simulink model "project_simu"  (R2019a)
settings: Solver=VariableStepAuto  StartTime=0.0  StopTime=1  RelTol=1e-3
values from neighbouring files (symbols this model uses):
  banks = 1e6*banks_data    [project.m]
  f = Filters/mean(Filters)    [project.m]
  lines = lines_data    [project.m]
  loads = zeros(10,2)    [project.m]
  m = 2    [project.m]
libraries: powerlib x87, powerlib_meascontrol x1, sps_avr x1
(part 1 of 2)
settings Model: OrderedModelArguments=off  Creator=jedevisscher  LastModifiedBy=dimit
settings SolverCC: ZeroCrossAlgorithm=Adaptive
settings DataIOCC: ExternalInput=out.S5  ReturnWorkspaceOutputs=off
settings DebuggingCC: IgnoredZcDiagnostic=none  UnconnectedInputMsg=none  UnconnectedOutputMsg=none  UnconnectedLineMsg=none
settings SimscapeCC: SimscapeLogType=all  SimscapeLogSimulationStatistics=on  SimscapeLogToSDI=on  SimscapeLogOpenViewer=on

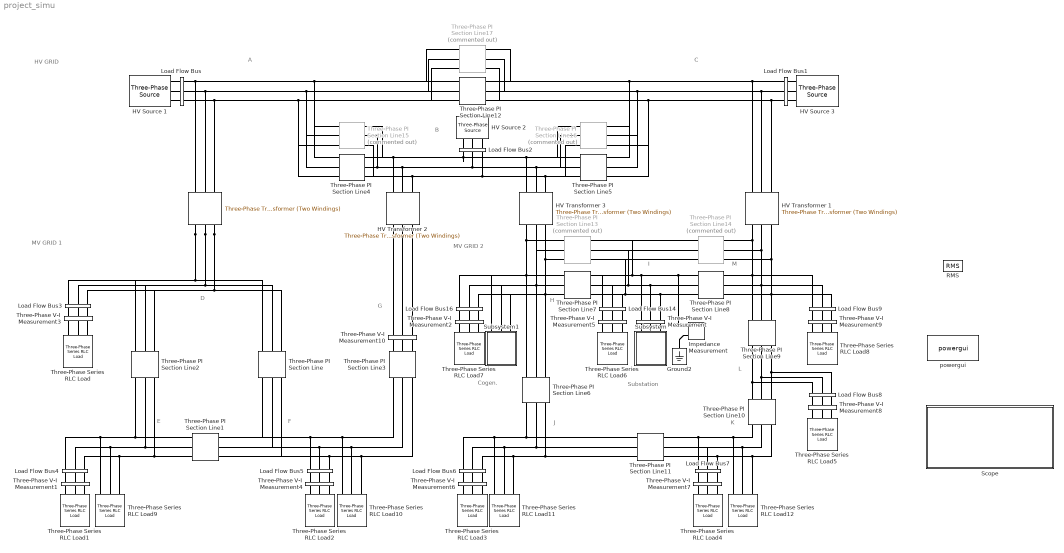
== system project_simu ==
  note: A
  note: B
  note: C
  note: D
  note: E
  note: F
  note: G
  note: H
  note: I
  note: J
  note: K
  note: L
  note: M
  note: HV GRID
  note: MV GRID 1
  note: MV GRID 2
  note: Substation
  note: Cogen.
  " " : powerlib/Elements/Three-Phase Transformer (Two Windings)  Winding1Connection=Yg  Winding2Connection=Yg  CoreType=Three single-phase transformers  SetSaturation=off  Hysteresis=off  DataFile='hysteresis'  SetInitialFlux=off  Measurements=None  UNITS=pu  NominalPower=[ 100e6 , 50 ]  Winding1=[220e3 0.002 0.08]  Winding2=[70e3 0.002 0.08]  Rm=500  Lm=500  L0=0.5  Saturation=[0 0;0.0024 1.2;0.99998 1.52]  InitialFluxes=[ 0.8 , -0.8 , 0.7 ]  BreakLoop=off  DiscreteSolver=Trapezoidal iterative  DataType=off  TransfoNumber=1
      settings: SourceProductName=Simscape Electrical
  Ground2 : powerlib/Elements/Ground  LConnTagsString=a
      settings: SourceProductName=Simscape Electrical
  HV Source 1 : powerlib/Electrical Sources/Three-Phase Source  InternalConnection=Yg  VoltagePhases=off  Voltage=220e3  PhaseAngle=0  Voltage_phases=[ 1.00409 1.00409 1.00409]*127017  PhaseAngles_phases=[ 1.18424 -118.816 121.184]  Frequency=50  NonIdealSource=on  SpecifyImpedance=on  Resistance=0  Inductance=0  ShortCircuitLevel=10e9  BaseVoltage=220e3  XRratio=7  BusType=swing  Pref=10e3  Qref=0  Prefabc=[3333.33 3333.33 3333.33]  Qrefabc=[0 0 0]  Qmin=-inf  Qmax=inf
      settings: SourceProductName=Simscape Electrical
  HV Source 2 : powerlib/Electrical Sources/Three-Phase Source  InternalConnection=Yg  VoltagePhases=off  Voltage=220e3  PhaseAngle=0  Voltage_phases=[ 1.01 1.01 1.01]*127017  PhaseAngles_phases=[ -2.01012 -122.01 117.99]  Frequency=50  NonIdealSource=on  SpecifyImpedance=on  Resistance=0  Inductance=0  ShortCircuitLevel=5e9  BaseVoltage=220e3  XRratio=6  BusType=PV  Pref=10e3  Qref=0  Prefabc=[3333.33 3333.33 3333.33]  Qrefabc=[0 0 0]  Qmin=-inf  Qmax=inf
      settings: SourceProductName=Simscape Electrical
  HV Source 3 : powerlib/Electrical Sources/Three-Phase Source  InternalConnection=Yg  VoltagePhases=off  Voltage=220e3  PhaseAngle=0  Voltage_phases=[ 1.01287 1.01287 1.01287]*127017  PhaseAngles_phases=[ -2.11617 -122.116 117.884]  Frequency=50  NonIdealSource=on  SpecifyImpedance=on  Resistance=0  Inductance=0  ShortCircuitLevel=3.5e9  BaseVoltage=220e3  XRratio=6  BusType=PV  Pref=10e3  Qref=0  Prefabc=[3333.33 3333.33 3333.33]  Qrefabc=[0 0 0]  Qmin=-inf  Qmax=inf
      settings: SourceProductName=Simscape Electrical
  HV Transformer 1 : powerlib/Elements/Three-Phase Transformer (Two Windings)  Winding1Connection=Yg  Winding2Connection=Yg  CoreType=Three single-phase transformers  SetSaturation=off  Hysteresis=off  DataFile='hysteresis'  SetInitialFlux=off  Measurements=None  UNITS=pu  NominalPower=[ 220e6 , 50 ]  Winding1=[220e3 0.001 0.1]  Winding2=[70e3 0.001 0.1]  Rm=500  Lm=500  L0=0.5  Saturation=[0 0;0.0024 1.2;0.99998 1.52]  InitialFluxes=[ 0.8 , -0.8 , 0.7 ]  BreakLoop=off  DiscreteSolver=Trapezoidal iterative  DataType=off  TransfoNumber=1
      settings: SourceProductName=Simscape Electrical
  HV Transformer 2 : powerlib/Elements/Three-Phase Transformer (Two Windings)  Winding1Connection=Yg  Winding2Connection=Yg  CoreType=Three single-phase transformers  SetSaturation=off  Hysteresis=off  DataFile='hysteresis'  SetInitialFlux=off  Measurements=None  UNITS=pu  NominalPower=[ 100e6 , 50 ]  Winding1=[220e3 0.002 0.075]  Winding2=[70e3 0.002 0.075]  Rm=500  Lm=500  L0=0.5  Saturation=[0 0;0.0024 1.2;0.99998 1.52]  InitialFluxes=[ 0.8 , -0.8 , 0.7 ]  BreakLoop=off  DiscreteSolver=Trapezoidal iterative  DataType=off  TransfoNumber=1
      settings: SourceProductName=Simscape Electrical
  HV Transformer 3 : powerlib/Elements/Three-Phase Transformer (Two Windings)  Winding1Connection=Yg  Winding2Connection=Yg  CoreType=Three single-phase transformers  SetSaturation=off  Hysteresis=off  DataFile='hysteresis'  SetInitialFlux=off  Measurements=None  UNITS=pu  NominalPower=[ 220e6 , 50 ]  Winding1=[220e3 0.001 0.1]  Winding2=[70e3 0.001 0.1]  Rm=500  Lm=500  L0=0.5  Saturation=[0 0;0.0024 1.2;0.99998 1.52]  InitialFluxes=[ 0.8 , -0.8 , 0.7 ]  BreakLoop=off  DiscreteSolver=Trapezoidal iterative  DataType=off  TransfoNumber=1
      settings: SourceProductName=Simscape Electrical
  Impedance Measurement : powerlib/Measurements/Impedance Measurement  LConnTagsString=+|-  Factor=1
      settings: SourceProductName=Simscape Electrical  SourceProductBaseCode=PS
  Load Flow Bus : powerlib/Measurements/Load Flow Bus  LConnTagsString=a|b|c  RConnTagsString=a|b|c  Phases=ABC  Connectors=on both sides  ID=BUS_A  Vbase=220e3/sqrt(3)  Vref=[1 1 1]  Vangle=[0 -120 120]  VLF=1  VLFb=1  VLFc=1  angleLF=0  angleLFb=-120  angleLFc=120
      settings: SourceProductName=Simscape Electrical
  Load Flow Bus1 : powerlib/Measurements/Load Flow Bus  LConnTagsString=a|b|c  RConnTagsString=a|b|c  Phases=ABC  Connectors=on both sides  ID=BUS_C  Vbase=220e3/sqrt(3)  Vref=[1 1 1]  Vangle=[0 -120 120]  VLF=1  VLFb=1  VLFc=1  angleLF=-1.995  angleLFb=-122  angleLFc=118
      settings: SourceProductName=Simscape Electrical
  Load Flow Bus14 : powerlib/Measurements/Load Flow Bus  LConnTagsString=a|b|c  RConnTagsString=a|b|c  Phases=ABC  Connectors=on both sides  ID=BUS_I  Vbase=70e3/sqrt(3)  Vref=[1 0 0]  Vangle=[0 -120 120]  VLF=0.9635  VLFb=0.9635  VLFc=0.9635  angleLF=-6.316  angleLFb=-126.3  angleLFc=113.7
      settings: SourceProductName=Simscape Electrical
  Load Flow Bus16 : powerlib/Measurements/Load Flow Bus  LConnTagsString=a|b|c  RConnTagsString=a|b|c  Phases=ABC  Connectors=on both sides  ID=BUS_H  Vbase=70e3/sqrt(3)  Vref=[1 1 1]  Vangle=[0 -120 120]  VLF=0.9665  VLFb=0.9665  VLFc=0.9665  angleLF=-6.129  angleLFb=-126.1  angleLFc=113.9
      settings: SourceProductName=Simscape Electrical
  Load Flow Bus2 : powerlib/Measurements/Load Flow Bus  LConnTagsString=a|b|c  RConnTagsString=a|b|c  Phases=ABC  Connectors=on both sides  ID=BUS_B  Vbase=220e3/sqrt(3)  Vref=[1 1 1]  Vangle=[0 -120 120]  VLF=1  VLFb=1  VLFc=1  angleLF=-1.916  angleLFb=-121.9  angleLFc=118.1
      settings: SourceProductName=Simscape Electrical
  Load Flow Bus3 : powerlib/Measurements/Load Flow Bus  LConnTagsString=a|b|c  RConnTagsString=a|b|c  Phases=ABC  Connectors=on both sides  ID=BUS_D  Vbase=70e3/sqrt(3)  Vref=[1 1 1]  Vangle=[0 -120 120]  VLF=0.9793  VLFb=0.9793  VLFc=0.9793  angleLF=-3.625  angleLFb=-123.6  angleLFc=116.4
      settings: SourceProductName=Simscape Electrical
  Load Flow Bus4 : powerlib/Measurements/Load Flow Bus  LConnTagsString=a|b|c  RConnTagsString=a|b|c  Phases=ABC  Connectors=on both sides  ID=BUS_E  Vbase=70e3/sqrt(3)  Vref=[1 1 1]  Vangle=[0 -120 120]  VLF=0.9694  VLFb=0.9694  VLFc=0.9694  angleLF=-4.52  angleLFb=-124.5  angleLFc=115.5
      settings: SourceProductName=Simscape Electrical
  Load Flow Bus5 : powerlib/Measurements/Load Flow Bus  LConnTagsString=a|b|c  RConnTagsString=a|b|c  Phases=ABC  Connectors=on both sides  ID=BUS_F  Vbase=70e3/sqrt(3)  Vref=[1 1 1]  Vangle=[0 -120 120]  VLF=0.972  VLFb=0.972  VLFc=0.972  angleLF=-4.299  angleLFb=-124.3  angleLFc=115.7
      settings: SourceProductName=Simscape Electrical
  Load Flow Bus6 : powerlib/Measurements/Load Flow Bus  LConnTagsString=a|b|c  RConnTagsString=a|b|c  Phases=ABC  Connectors=on both sides  ID=BUS_J  Vbase=70e3/sqrt(3)  Vref=[1 1 1]  Vangle=[0 4/3*pi 2/3*pi]  VLF=0.9323  VLFb=0.9323  VLFc=0.9323  angleLF=-9.193  angleLFb=-129.2  angleLFc=110.8
      settings: SourceProductName=Simscape Electrical
  Load Flow Bus7 : powerlib/Measurements/Load Flow Bus  LConnTagsString=a|b|c  RConnTagsString=a|b|c  Phases=ABC  Connectors=on both sides  ID=BUS_K  Vbase=70e3/sqrt(3)  Vref=[1 1 1]  Vangle=[0 -120 120]  VLF=0.9399  VLFb=0.9399  VLFc=0.9399  angleLF=-8.17  angleLFb=-128.2  angleLFc=111.8
      settings: SourceProductName=Simscape Electrical
  Load Flow Bus8 : powerlib/Measurements/Load Flow Bus  LConnTagsString=a|b|c  RConnTagsString=a|b|c  Phases=ABC  Connectors=on both sides  ID=BUS_L  Vbase=70e3/sqrt(3)  Vref=[1 1 1]  Vangle=[0 -120 120]  VLF=0.944  VLFb=0.944  VLFc=0.944  angleLF=-7.8  angleLFb=-127.8  angleLFc=112.2
      settings: SourceProductName=Simscape Electrical
  Load Flow Bus9 : powerlib/Measurements/Load Flow Bus  LConnTagsString=a|b|c  RConnTagsString=a|b|c  Phases=ABC  Connectors=on both sides  ID=BUS_M  Vbase=70e3/sqrt(3)  Vref=[1 1 1]  Vangle=[0 -120 120]  VLF=0.9654  VLFb=0.9654  VLFc=0.9654  angleLF=-6.231  angleLFb=-126.2  angleLFc=113.8
      settings: SourceProductName=Simscape Electrical
  RMS : powerlib_meascontrol/Measurements/RMS  TrueRMS=on  Freq=50  RMSInit=120  Ts=0
      settings: SourceProductName=Simscape Electrical
  Scope : Subsystem
  Subsystem : Subsystem
  Subsystem1 : Subsystem
  Three-Phase PI Section Line : powerlib/Elements/Three-Phase PI Section Line  LConnTagsString=a|b|c  RConnTagsString=A|B|C  Frequency=50  Resistances=[lines(5,1) lines(5,2)]  Inductances=[lines(5,3) lines(5,4)]  Capacitances=[lines(5,5) lines(5,6)]  Length=lines(5,7)
      settings: SourceProductName=Simscape Electrical
  Three-Phase PI Section Line1 : powerlib/Elements/Three-Phase PI Section Line  LConnTagsString=a|b|c  RConnTagsString=A|B|C  Frequency=50  Resistances=[lines(6,1) lines(6,2)]  Inductances=[lines(6,3) lines(6,4)]  Capacitances=[lines(6,5) lines(6,6)]  Length=lines(6,7)
      settings: SourceProductName=Simscape Electrical
  Three-Phase PI Section Line10 : powerlib/Elements/Three-Phase PI Section Line  LConnTagsString=a|b|c  RConnTagsString=A|B|C  Frequency=50  Resistances=[lines(12,1) lines(12,2)]  Inductances=[lines(12,3) lines(12,4)]  Capacitances=[lines(12,5) lines(12,6)]  Length=lines(12,7)
      settings: SourceProductName=Simscape Electrical
  Three-Phase PI Section Line11 : powerlib/Elements/Three-Phase PI Section Line  LConnTagsString=a|b|c  RConnTagsString=A|B|C  Frequency=50  Resistances=[lines(13,1) lines(13,2)]  Inductances=[lines(13,3) lines(13,4)]  Capacitances=[lines(13,5) lines(13,6)]  Length=lines(13,7)
      settings: SourceProductName=Simscape Electrical
  Three-Phase PI Section Line12 : powerlib/Elements/Three-Phase PI Section Line  LConnTagsString=a|b|c  RConnTagsString=A|B|C  Frequency=50  Resistances=[lines(2,1) lines(2,2)]  Inductances=[lines(2,3) lines(2,4)]  Capacitances=[lines(2,5) lines(2,6)]  Length=lines(2,7)
      settings: SourceProductName=Simscape Electrical
  Three-Phase PI Section Line13 : powerlib/Elements/Three-Phase PI Section Line  Commented=on  LConnTagsString=a|b|c  RConnTagsString=A|B|C  Frequency=50  Resistances=[lines(9,1) lines(9,2)]  Inductances=[lines(9,3) lines(9,4)]  Capacitances=[lines(9,5) lines(9,6)]  Length=lines(9,7)
      settings: SourceProductName=Simscape Electrical
  Three-Phase PI Section Line14 : powerlib/Elements/Three-Phase PI Section Line  Commented=on  LConnTagsString=a|b|c  RConnTagsString=A|B|C  Frequency=50  Resistances=[lines(10,1) lines(10,2)]  Inductances=[lines(10,3) lines(10,4)]  Capacitances=[lines(10,5) lines(10,6)]  Length=lines(10,7)
      settings: SourceProductName=Simscape Electrical
  Three-Phase PI Section Line15 : powerlib/Elements/Three-Phase PI Section Line  Commented=on  LConnTagsString=a|b|c  RConnTagsString=A|B|C  Frequency=50  Resistances=[lines(1,1) lines(1,2)]  Inductances=[lines(1,3) lines(1,4)]  Capacitances=[lines(1,5) lines(1,6)]  Length=lines(1,7)
      settings: SourceProductName=Simscape Electrical
  Three-Phase PI Section Line16 : powerlib/Elements/Three-Phase PI Section Line  Commented=on  LConnTagsString=a|b|c  RConnTagsString=A|B|C  Frequency=50  Resistances=[lines(3,1) lines(3,2)]  Inductances=[lines(3,3) lines(3,4)]  Capacitances=[lines(3,5) lines(3,6)]  Length=lines(3,7)
      settings: SourceProductName=Simscape Electrical
  Three-Phase PI Section Line17 : powerlib/Elements/Three-Phase PI Section Line  Commented=on  LConnTagsString=a|b|c  RConnTagsString=A|B|C  Frequency=50  Resistances=[lines(2,1) lines(2,2)]  Inductances=[lines(2,3) lines(2,4)]  Capacitances=[lines(2,5) lines(2,6)]  Length=lines(2,7)
      settings: SourceProductName=Simscape Electrical
  Three-Phase PI Section Line2 : powerlib/Elements/Three-Phase PI Section Line  LConnTagsString=a|b|c  RConnTagsString=A|B|C  Frequency=50  Resistances=[lines(4,1) lines(4,2)]  Inductances=[lines(4,3) lines(4,4)]  Capacitances=[lines(4,5) lines(4,6)]  Length=lines(4,7)
      settings: SourceProductName=Simscape Electrical
  Three-Phase PI Section Line3 : powerlib/Elements/Three-Phase PI Section Line  LConnTagsString=a|b|c  RConnTagsString=A|B|C  Frequency=50  Resistances=[lines(7,1) lines(7,2)]  Inductances=[lines(7,3) lines(7,4)]  Capacitances=[lines(7,5) lines(7,6)]  Length=lines(7,7)
      settings: SourceProductName=Simscape Electrical
  Three-Phase PI Section Line4 : powerlib/Elements/Three-Phase PI Section Line  LConnTagsString=a|b|c  RConnTagsString=A|B|C  Frequency=50  Resistances=[lines(1,1) lines(1,2)]  Inductances=[lines(1,3) lines(1,4)]  Capacitances=[lines(1,5) lines(1,6)]  Length=lines(1,7)
      settings: SourceProductName=Simscape Electrical
  Three-Phase PI Section Line5 : powerlib/Elements/Three-Phase PI Section Line  LConnTagsString=a|b|c  RConnTagsString=A|B|C  Frequency=50  Resistances=[lines(3,1) lines(3,2)]  Inductances=[lines(3,3) lines(3,4)]  Capacitances=[lines(3,5) lines(3,6)]  Length=lines(3,7)
      settings: SourceProductName=Simscape Electrical
  Three-Phase PI Section Line6 : powerlib/Elements/Three-Phase PI Section Line  LConnTagsString=a|b|c  RConnTagsString=A|B|C  Frequency=50  Resistances=[lines(8,1) lines(8,2)]  Inductances=[lines(8,3) lines(8,4)]  Capacitances=[lines(8,5) lines(8,6)]  Length=lines(8,7)
      settings: SourceProductName=Simscape Electrical
  Three-Phase PI Section Line7 : powerlib/Elements/Three-Phase PI Section Line  LConnTagsString=a|b|c  RConnTagsString=A|B|C  Frequency=50  Resistances=[lines(9,1) lines(9,2)]  Inductances=[lines(9,3) lines(9,4)]  Capacitances=[lines(9,5) lines(9,6)]  Length=lines(9,7)
      settings: SourceProductName=Simscape Electrical
  Three-Phase PI Section Line8 : powerlib/Elements/Three-Phase PI Section Line  LConnTagsString=a|b|c  RConnTagsString=A|B|C  Frequency=50  Resistances=[lines(10,1) lines(10,2)]  Inductances=[lines(10,3) lines(10,4)]  Capacitances=[lines(10,5) lines(10,6)]  Length=lines(10,7)
      settings: SourceProductName=Simscape Electrical
  Three-Phase PI Section Line9 : powerlib/Elements/Three-Phase PI Section Line  LConnTagsString=a|b|c  RConnTagsString=A|B|C  Frequency=50  Resistances=[lines(11,1) lines(11,2)]  Inductances=[lines(11,3) lines(11,4)]  Capacitances=[lines(11,5) lines(11,6)]  Length=lines(11,7)
      settings: SourceProductName=Simscape Electrical
  Three-Phase Series RLC Load : powerlib/Elements/Three-Phase Series RLC Load  LConnTagsString=A|B|C  Configuration=Y (grounded)  NominalVoltage=70e3  Vabc=[ 0.979308 0.979308 0.979307]*40414.5  Vabcp=[1e3 1e3 1e3]  NominalFrequency=50  UnbalancedPower=off  ActivePower=loads(1,1)  InductivePower=loads(1,2)  CapacitivePower=0  Pabc=[10e3 9e3 11e3]  QLabc=[100 90 110]  QCabc=[100 90 110]  Pabcp=[10e3 9e3 11e3]  QLabcp=[100 90 110]  QCabcp=[100 90 110]  Measurements=None  LoadType=constant PQ
      settings: SourceProductName=Simscape Electrical
  Three-Phase Series RLC Load1 : powerlib/Elements/Three-Phase Series RLC Load  LConnTagsString=A|B|C  Configuration=Y (grounded)  NominalVoltage=70e3  Vabc=[1e3 1e3 1e3]  Vabcp=[1e3 1e3 1e3]  NominalFrequency=50  UnbalancedPower=off  ActivePower=loads(2,1)  InductivePower=loads(2,2)  CapacitivePower=0  Pabc=[10e3 9e3 11e3]  QLabc=[100 90 110]  QCabc=[100 90 110]  Pabcp=[10e3 9e3 11e3]  QLabcp=[100 90 110]  QCabcp=[100 90 110]  Measurements=None  LoadType=constant PQ
      settings: SourceProductName=Simscape Electrical
  Three-Phase Series RLC Load10 : powerlib/Elements/Three-Phase Series RLC Load  LConnTagsString=A|B|C  Configuration=Y (grounded)  NominalVoltage=70e3  Vabc=[1e3 1e3 1e3]  Vabcp=[1e3 1e3 1e3]  NominalFrequency=50  UnbalancedPower=off  ActivePower=0  InductivePower=0  CapacitivePower=banks(2,m)  Pabc=[10e3 9e3 11e3]  QLabc=[100 90 110]  QCabc=[100 90 110]  Pabcp=[10e3 9e3 11e3]  QLabcp=[100 90 110]  QCabcp=[100 90 110]  Measurements=None  LoadType=constant PQ
      settings: SourceProductName=Simscape Electrical
  Three-Phase Series RLC Load11 : powerlib/Elements/Three-Phase Series RLC Load  LConnTagsString=A|B|C  Configuration=Y (grounded)  NominalVoltage=70e3  Vabc=[1e3 1e3 1e3]  Vabcp=[1e3 1e3 1e3]  NominalFrequency=50  UnbalancedPower=off  ActivePower=0  InductivePower=0  CapacitivePower=banks(3,m)  Pabc=[10e3 9e3 11e3]  QLabc=[100 90 110]  QCabc=[100 90 110]  Pabcp=[10e3 9e3 11e3]  QLabcp=[100 90 110]  QCabcp=[100 90 110]  Measurements=None  LoadType=constant PQ
      settings: SourceProductName=Simscape Electrical
  Three-Phase Series RLC Load12 : powerlib/Elements/Three-Phase Series RLC Load  LConnTagsString=A|B|C  Configuration=Y (grounded)  NominalVoltage=70e3  Vabc=[1e3 1e3 1e3]  Vabcp=[1e3 1e3 1e3]  NominalFrequency=50  UnbalancedPower=off  ActivePower=0  InductivePower=0  CapacitivePower=banks(4,m)  Pabc=[10e3 9e3 11e3]  QLabc=[100 90 110]  QCabc=[100 90 110]  Pabcp=[10e3 9e3 11e3]  QLabcp=[100 90 110]  QCabcp=[100 90 110]  Measurements=None  LoadType=constant PQ
      settings: SourceProductName=Simscape Electrical
  Three-Phase Series RLC Load2 : powerlib/Elements/Three-Phase Series RLC Load  LConnTagsString=A|B|C  Configuration=Y (grounded)  NominalVoltage=70e3  Vabc=[1e3 1e3 1e3]  Vabcp=[1e3 1e3 1e3]  NominalFrequency=50  UnbalancedPower=off  ActivePower=loads(3,1)  InductivePower=loads(3,2)  CapacitivePower=0  Pabc=[10e3 9e3 11e3]  QLabc=[100 90 110]  QCabc=[100 90 110]  Pabcp=[10e3 9e3 11e3]  QLabcp=[100 90 110]  QCabcp=[100 90 110]  Measurements=None  LoadType=constant PQ
      settings: SourceProductName=Simscape Electrical
  Three-Phase Series RLC Load3 : powerlib/Elements/Three-Phase Series RLC Load  LConnTagsString=A|B|C  Configuration=Y (grounded)  NominalVoltage=70e3  Vabc=[1e3 1e3 1e3]  Vabcp=[1e3 1e3 1e3]  NominalFrequency=50  UnbalancedPower=off  ActivePower=loads(6,1)  InductivePower=loads(6,2)  CapacitivePower=0  Pabc=[10e3 9e3 11e3]  QLabc=[100 90 110]  QCabc=[100 90 110]  Pabcp=[10e3 9e3 11e3]  QLabcp=[100 90 110]  QCabcp=[100 90 110]  Measurements=None  LoadType=constant PQ
      settings: SourceProductName=Simscape Electrical
  Three-Phase Series RLC Load4 : powerlib/Elements/Three-Phase Series RLC Load  LConnTagsString=A|B|C  Configuration=Y (grounded)  NominalVoltage=70e3  Vabc=[1e3 1e3 1e3]  Vabcp=[1e3 1e3 1e3]  NominalFrequency=50  UnbalancedPower=off  ActivePower=loads(7,1)  InductivePower=loads(7,2)  CapacitivePower=0  Pabc=[10e3 9e3 11e3]  QLabc=[100 90 110]  QCabc=[100 90 110]  Pabcp=[10e3 9e3 11e3]  QLabcp=[100 90 110]  QCabcp=[100 90 110]  Measurements=None  LoadType=constant PQ
      settings: SourceProductName=Simscape Electrical
  Three-Phase Series RLC Load5 : powerlib/Elements/Three-Phase Series RLC Load  LConnTagsString=A|B|C  Configuration=Y (grounded)  NominalVoltage=70e3  Vabc=[1e3 1e3 1e3]  Vabcp=[1e3 1e3 1e3]  NominalFrequency=50  UnbalancedPower=off  ActivePower=loads(8,1)  InductivePower=loads(8,2)  CapacitivePower=0  Pabc=[10e3 9e3 11e3]  QLabc=[100 90 110]  QCabc=[100 90 110]  Pabcp=[10e3 9e3 11e3]  QLabcp=[100 90 110]  QCabcp=[100 90 110]  Measurements=None  LoadType=constant PQ
      settings: SourceProductName=Simscape Electrical
  Three-Phase Series RLC Load6 : powerlib/Elements/Three-Phase Series RLC Load  LConnTagsString=A|B|C  Configuration=Y (grounded)  NominalVoltage=70e3  Vabc=[1e3 1e3 1e3]  Vabcp=[1e3 1e3 1e3]  NominalFrequency=50  UnbalancedPower=off  ActivePower=loads(5,1)  InductivePower=loads(5,2)  CapacitivePower=0  Pabc=[10e3 9e3 11e3]  QLabc=[100 90 110]  QCabc=[100 90 110]  Pabcp=[10e3 9e3 11e3]  QLabcp=[100 90 110]  QCabcp=[100 90 110]  Measurements=None  LoadType=constant PQ
      settings: SourceProductName=Simscape Electrical
  Three-Phase Series RLC Load7 : powerlib/Elements/Three-Phase Series RLC Load  LConnTagsString=A|B|C  Configuration=Y (grounded)  NominalVoltage=70e3  Vabc=[1e3 1e3 1e3]  Vabcp=[1e3 1e3 1e3]  NominalFrequency=50  UnbalancedPower=off  ActivePower=loads(4,1)  InductivePower=loads(4,2)  CapacitivePower=0  Pabc=[10e3 9e3 11e3]  QLabc=[100 90 110]  QCabc=[100 90 110]  Pabcp=[10e3 9e3 11e3]  QLabcp=[100 90 110]  QCabcp=[100 90 110]  Measurements=None  LoadType=constant PQ
      settings: SourceProductName=Simscape Electrical
  Three-Phase Series RLC Load8 : powerlib/Elements/Three-Phase Series RLC Load  LConnTagsString=A|B|C  Configuration=Y (grounded)  NominalVoltage=70e3  Vabc=[1e3 1e3 1e3]  Vabcp=[1e3 1e3 1e3]  NominalFrequency=50  UnbalancedPower=off  ActivePower=loads(9,1)  InductivePower=loads(9,2)  CapacitivePower=0  Pabc=[10e3 9e3 11e3]  QLabc=[100 90 110]  QCabc=[100 90 110]  Pabcp=[10e3 9e3 11e3]  QLabcp=[100 90 110]  QCabcp=[100 90 110]  Measurements=None  LoadType=constant PQ
      settings: SourceProductName=Simscape Electrical
  Three-Phase Series RLC Load9 : powerlib/Elements/Three-Phase Series RLC Load  LConnTagsString=A|B|C  Configuration=Y (grounded)  NominalVoltage=70e3  Vabc=[1e3 1e3 1e3]  Vabcp=[1e3 1e3 1e3]  NominalFrequency=50  UnbalancedPower=off  ActivePower=0  InductivePower=0  CapacitivePower=banks(1,m)  Pabc=[10e3 9e3 11e3]  QLabc=[100 90 110]  QCabc=[100 90 110]  Pabcp=[10e3 9e3 11e3]  QLabcp=[100 90 110]  QCabcp=[100 90 110]  Measurements=None  LoadType=constant PQ
      settings: SourceProductName=Simscape Electrical
  Three-Phase V-I Measurement : powerlib/Measurements/Three-Phase V-I Measurement  VoltageMeasurement=phase-to-ground  SetLabelV=on  LabelV=Vpcc  Vpu=on  VpuLL=off  CurrentMeasurement=yes  SetLabelI=on  LabelI=Ipcc  Ipu=on  Pbase=220e6  Vbase=70e3  OutputType=Complex  PhasorSimulation=off  PSBequivalent=0
      settings: SourceProductName=Simscape Electrical
  Three-Phase V-I Measurement1 : powerlib/Measurements/Three-Phase V-I Measurement  VoltageMeasurement=phase-to-ground  SetLabelV=on  LabelV=VE  Vpu=on  VpuLL=off  CurrentMeasurement=yes  SetLabelI=on  LabelI=IE  Ipu=on  Pbase=100e6  Vbase=70e3  OutputType=Complex  PhasorSimulation=off  PSBequivalent=0
      settings: SourceProductName=Simscape Electrical
  Three-Phase V-I Measurement10 : powerlib/Measurements/Three-Phase V-I Measurement  VoltageMeasurement=phase-to-ground  SetLabelV=on  LabelV=VG  Vpu=on  VpuLL=off  CurrentMeasurement=yes  SetLabelI=on  LabelI=IG  Ipu=on  Pbase=100e6  Vbase=70e3  OutputType=Complex  PhasorSimulation=off  PSBequivalent=0
      settings: SourceProductName=Simscape Electrical
  Three-Phase V-I Measurement2 : powerlib/Measurements/Three-Phase V-I Measurement  VoltageMeasurement=phase-to-ground  SetLabelV=on  LabelV=VH  Vpu=on  VpuLL=off  CurrentMeasurement=yes  SetLabelI=on  LabelI=IH  Ipu=on  Pbase=220e6  Vbase=70e3  OutputType=Complex  PhasorSimulation=off  PSBequivalent=0
      settings: SourceProductName=Simscape Electrical
  Three-Phase V-I Measurement3 : powerlib/Measurements/Three-Phase V-I Measurement  VoltageMeasurement=phase-to-ground  SetLabelV=on  LabelV=VD  Vpu=on  VpuLL=off  CurrentMeasurement=yes  SetLabelI=on  LabelI=ID  Ipu=on  Pbase=100e6  Vbase=70e3  OutputType=Complex  PhasorSimulation=off  PSBequivalent=0
      settings: SourceProductName=Simscape Electrical
  Three-Phase V-I Measurement4 : powerlib/Measurements/Three-Phase V-I Measurement  VoltageMeasurement=phase-to-ground  SetLabelV=on  LabelV=VF  Vpu=on  VpuLL=off  CurrentMeasurement=yes  SetLabelI=on  LabelI=IF  Ipu=on  Pbase=100e6  Vbase=70e3  OutputType=Complex  PhasorSimulation=off  PSBequivalent=0
      settings: SourceProductName=Simscape Electrical
  Three-Phase V-I Measurement5 : powerlib/Measurements/Three-Phase V-I Measurement  VoltageMeasurement=phase-to-ground  SetLabelV=on  LabelV=VI  Vpu=on  VpuLL=off  CurrentMeasurement=yes  SetLabelI=on  LabelI=II  Ipu=on  Pbase=220e6  Vbase=70e3  OutputType=Complex  PhasorSimulation=off  PSBequivalent=0
      settings: SourceProductName=Simscape Electrical
  Three-Phase V-I Measurement6 : powerlib/Measurements/Three-Phase V-I Measurement  VoltageMeasurement=phase-to-ground  SetLabelV=on  LabelV=VJ  Vpu=on  VpuLL=off  CurrentMeasurement=yes  SetLabelI=on  LabelI=IJ  Ipu=on  Pbase=220e6  Vbase=70e3  OutputType=Complex  PhasorSimulation=off  PSBequivalent=0
      settings: SourceProductName=Simscape Electrical
  Three-Phase V-I Measurement7 : powerlib/Measurements/Three-Phase V-I Measurement  VoltageMeasurement=phase-to-ground  SetLabelV=on  LabelV=VK  Vpu=on  VpuLL=off  CurrentMeasurement=yes  SetLabelI=on  LabelI=IK  Ipu=on  Pbase=220e6  Vbase=70e3  OutputType=Complex  PhasorSimulation=off  PSBequivalent=0
      settings: SourceProductName=Simscape Electrical
  Three-Phase V-I Measurement8 : powerlib/Measurements/Three-Phase V-I Measurement  VoltageMeasurement=phase-to-ground  SetLabelV=on  LabelV=VL  Vpu=on  VpuLL=off  CurrentMeasurement=yes  SetLabelI=on  LabelI=IL  Ipu=on  Pbase=220e6  Vbase=70e3  OutputType=Complex  PhasorSimulation=off  PSBequivalent=0
      settings: SourceProductName=Simscape Electrical
  Three-Phase V-I Measurement9 : powerlib/Measurements/Three-Phase V-I Measurement  VoltageMeasurement=phase-to-ground  SetLabelV=on  LabelV=VM  Vpu=on  VpuLL=off  CurrentMeasurement=yes  SetLabelI=on  LabelI=IM  Ipu=on  Pbase=220e6  Vbase=70e3  OutputType=Complex  PhasorSimulation=off  PSBequivalent=0
      settings: SourceProductName=Simscape Electrical
  powergui : powerlib/powergui  Priority=1  SimulationMode=Discrete  SampleTime=1e-5  frequency=50  Iterations=50  frequencyindice=60  Pbase=100e6  ErrMax=1e-4  UnitsV=kV  UnitsW=MW  buscounter=0  FunctionMessages=off  echomessages=off  EnableUseOfTLC=off  CurrentSourceSwitches=off  DisableSnubberDevices=off  DisableRonSwitches=off  DisableVfSwitches=off  DisplayEquations=off  AutomaticDiscreteSolvers=off  SolverType=Tustin/Backward Euler (TBE)  Interpol=off  ExternalGateDelay=off  methode=off  Ts=100  x0status=blocks  SPID=on  SwTol=0  HookPort=off  NonlinearTolerance=0  nMaxIteration=15  ContinueOnMaxIteration=off  RestoreLinks=warning  ResistiveCurrentMeasurement=off  Frange=[0:1:1500]  Ylog=off  Xlog=off  ShowGrid=on  save=on  variable=Z2_f591122  structure=PCC  ZoomFFT=off  StartTime=0.1  cycles=45  DisplayStyle=1  fundamental=50  FreqAxis=on  MaxFrequency=2500  frequencyindicesteady=50  RmsSteady=2  display=off
      settings: SourceProductName=Simscape Electrical
  connections:
  Load Flow Bus/LConn1 -- HV Source 1/RConn1
  Load Flow Bus/RConn3 -- Three-Phase PI Section Line17/LConn3 -- Three-Phase PI Section Line12/LConn3 -- Three-Phase PI Section Line4/LConn3 -- Three-Phase PI Section Line15/LConn3 -- " "/LConn3
  Load Flow Bus/LConn2 -- HV Source 1/RConn2
  Load Flow Bus1/LConn1 -- HV Transformer 1/LConn1 -- Three-Phase PI Section Line17/RConn1 -- Three-Phase PI Section Line12/RConn1 -- Three-Phase PI Section Line5/RConn1 -- Three-Phase PI Section Line16/RConn1
  Load Flow Bus1/LConn3 -- HV Transformer 1/LConn3 -- Three-Phase PI Section Line17/RConn3 -- Three-Phase PI Section Line12/RConn3 -- Three-Phase PI Section Line5/RConn3 -- Three-Phase PI Section Line16/RConn3
  Load Flow Bus1/LConn2 -- HV Transformer 1/LConn2 -- Three-Phase PI Section Line17/RConn2 -- Three-Phase PI Section Line12/RConn2 -- Three-Phase PI Section Line16/RConn2 -- Three-Phase PI Section Line5/RConn2
  Three-Phase PI Section Line4/RConn2 -- Three-Phase PI Section Line15/RConn2 -- Load Flow Bus2/RConn2 -- Three-Phase PI Section Line16/LConn2 -- Three-Phase PI Section Line5/LConn2 -- HV Transformer 3/LConn2 -- HV Transformer 2/LConn2
  Three-Phase PI Section Line1/RConn1 -- Three-Phase PI Section Line/RConn1 -- Three-Phase PI Section Line3/LConn1 -- Three-Phase Series RLC Load10/LConn1 -- Load Flow Bus5/LConn1
  Three-Phase PI Section Line1/RConn2 -- Three-Phase PI Section Line/RConn2 -- Three-Phase PI Section Line3/LConn2 -- Three-Phase Series RLC Load10/LConn2 -- Load Flow Bus5/LConn2
  Three-Phase PI Section Line1/RConn3 -- Three-Phase PI Section Line/RConn3 -- Three-Phase PI Section Line3/LConn3 -- Three-Phase Series RLC Load10/LConn3 -- Load Flow Bus5/LConn3
  " "/RConn1 -- Load Flow Bus3/LConn1 -- Three-Phase PI Section Line2/RConn1 -- Three-Phase PI Section Line/LConn1
  " "/RConn2 -- Load Flow Bus3/LConn2 -- Three-Phase PI Section Line2/RConn2 -- Three-Phase PI Section Line/LConn2
  " "/RConn3 -- Load Flow Bus3/LConn3 -- Three-Phase PI Section Line2/RConn3 -- Three-Phase PI Section Line/LConn3
  Load Flow Bus7/LConn1 -- Three-Phase PI Section Line11/RConn1 -- Three-Phase PI Section Line10/LConn1 -- Three-Phase Series RLC Load12/LConn1
  Load Flow Bus7/LConn3 -- Three-Phase PI Section Line11/RConn3 -- Three-Phase PI Section Line10/LConn3 -- Three-Phase Series RLC Load12/LConn3
  Three-Phase PI Section Line10/LConn2 -- Three-Phase PI Section Line11/RConn2 -- Load Flow Bus7/LConn2 -- Three-Phase Series RLC Load12/LConn2
  Three-Phase Series RLC Load11/LConn2 -- Load Flow Bus6/LConn2 -- Three-Phase PI Section Line11/LConn2 -- Three-Phase PI Section Line6/LConn2
  Three-Phase PI Section Line8/LConn3 -- Three-Phase PI Section Line14/LConn3 -- Three-Phase PI Section Line13/RConn3 -- Three-Phase PI Section Line7/RConn3 -- Load Flow Bus14/LConn3 -- Three-Phase V-I Measurement/LConn3
  HV Transformer 3/RConn1 -- Load Flow Bus16/LConn1 -- Subsystem1/RConn1 -- Three-Phase PI Section Line7/LConn1 -- Three-Phase PI Section Line6/RConn1 -- Three-Phase PI Section Line13/LConn1
  HV Transformer 3/RConn3 -- Three-Phase PI Section Line13/LConn3 -- Three-Phase PI Section Line7/LConn3 -- Load Flow Bus16/LConn3 -- Subsystem1/RConn3 -- Three-Phase PI Section Line6/RConn3
  Load Flow Bus8/LConn1 -- Three-Phase PI Section Line10/RConn1 -- Three-Phase PI Section Line9/LConn1
  Load Flow Bus8/LConn2 -- Three-Phase PI Section Line10/RConn2 -- Three-Phase PI Section Line9/LConn2
  Load Flow Bus8/LConn3 -- Three-Phase PI Section Line10/RConn3 -- Three-Phase PI Section Line9/LConn3
  HV Transformer 1/RConn1 -- Three-Phase PI Section Line14/RConn1 -- Three-Phase PI Section Line9/RConn1 -- Three-Phase PI Section Line8/RConn1 -- Load Flow Bus9/LConn1
  HV Transformer 1/RConn2 -- Three-Phase PI Section Line14/RConn2 -- Three-Phase PI Section Line9/RConn2 -- Three-Phase PI Section Line8/RConn2 -- Load Flow Bus9/LConn2
  Three-Phase Series RLC Load9/LConn1 -- Three-Phase PI Section Line1/LConn1 -- Three-Phase PI Section Line2/LConn1 -- Load Flow Bus4/LConn1
  Three-Phase Series RLC Load9/LConn2 -- Three-Phase PI Section Line1/LConn2 -- Three-Phase PI Section Line2/LConn2 -- Load Flow Bus4/LConn2
  Three-Phase Series RLC Load9/LConn3 -- Three-Phase PI Section Line2/LConn3 -- Three-Phase PI Section Line1/LConn3 -- Load Flow Bus4/LConn3
  Three-Phase Series RLC Load11/LConn1 -- Load Flow Bus6/LConn1 -- Three-Phase PI Section Line11/LConn1 -- Three-Phase PI Section Line6/LConn1
  Three-Phase Series RLC Load11/LConn3 -- Load Flow Bus6/LConn3 -- Three-Phase PI Section Line11/LConn3 -- Three-Phase PI Section Line6/LConn3
  HV Transformer 1/RConn3 -- Three-Phase PI Section Line14/RConn3 -- Three-Phase PI Section Line9/RConn3 -- Three-Phase PI Section Line8/RConn3 -- Load Flow Bus9/LConn3
  Three-Phase V-I Measurement/RConn1 -- Subsystem/LConn1
  Three-Phase V-I Measurement/RConn2 -- Subsystem/LConn2
  Subsystem/LConn3 -- Three-Phase V-I Measurement/RConn3
  Three-Phase Series RLC Load1/LConn1 -- Three-Phase V-I Measurement1/RConn1
  Three-Phase Series RLC Load1/LConn2 -- Three-Phase V-I Measurement1/RConn2
  Three-Phase Series RLC Load1/LConn3 -- Three-Phase V-I Measurement1/RConn3
  Three-Phase V-I Measurement2/RConn3 -- Three-Phase Series RLC Load7/LConn3
  Three-Phase V-I Measurement2/RConn2 -- Three-Phase Series RLC Load7/LConn2
  Three-Phase V-I Measurement2/RConn1 -- Three-Phase Series RLC Load7/LConn1
  Three-Phase V-I Measurement3/RConn1 -- Three-Phase Series RLC Load/LConn1
  Three-Phase V-I Measurement3/RConn2 -- Three-Phase Series RLC Load/LConn2
  Three-Phase V-I Measurement3/RConn3 -- Three-Phase Series RLC Load/LConn3
  Three-Phase V-I Measurement4/RConn1 -- Three-Phase Series RLC Load2/LConn1
  Three-Phase V-I Measurement4/RConn2 -- Three-Phase Series RLC Load2/LConn2
  Three-Phase V-I Measurement4/RConn3 -- Three-Phase Series RLC Load2/LConn3
  Three-Phase V-I Measurement5/RConn1 -- Three-Phase Series RLC Load6/LConn1
  Three-Phase V-I Measurement5/RConn2 -- Three-Phase Series RLC Load6/LConn2
  Three-Phase V-I Measurement5/RConn3 -- Three-Phase Series RLC Load6/LConn3
  Three-Phase V-I Measurement6/RConn1 -- Three-Phase Series RLC Load3/LConn1
  Three-Phase V-I Measurement6/RConn2 -- Three-Phase Series RLC Load3/LConn2
  Three-Phase V-I Measurement6/RConn3 -- Three-Phase Series RLC Load3/LConn3
  Three-Phase V-I Measurement7/RConn1 -- Three-Phase Series RLC Load4/LConn1
  Three-Phase V-I Measurement7/RConn2 -- Three-Phase Series RLC Load4/LConn2
  Three-Phase V-I Measurement7/RConn3 -- Three-Phase Series RLC Load4/LConn3
  Three-Phase V-I Measurement8/RConn1 -- Three-Phase Series RLC Load5/LConn1
  Three-Phase V-I Measurement8/RConn2 -- Three-Phase Series RLC Load5/LConn2
  Three-Phase V-I Measurement8/RConn3 -- Three-Phase Series RLC Load5/LConn3
  Three-Phase V-I Measurement9/RConn1 -- Three-Phase Series RLC Load8/LConn1
  Three-Phase V-I Measurement9/RConn2 -- Three-Phase Series RLC Load8/LConn2
  Three-Phase V-I Measurement9/RConn3 -- Three-Phase Series RLC Load8/LConn3
  Load Flow Bus1/RConn1 -- HV Source 3/RConn1
  Load Flow Bus1/RConn2 -- HV Source 3/RConn2
  Load Flow Bus1/RConn3 -- HV Source 3/RConn3
  Load Flow Bus2/LConn3 -- HV Source 2/RConn3
  HV Transformer 3/LConn3 -- Three-Phase PI Section Line16/LConn3 -- Three-Phase PI Section Line5/LConn3 -- Three-Phase PI Section Line15/RConn3 -- Three-Phase PI Section Line4/RConn3 -- HV Transformer 2/LConn3 -- Load Flow Bus2/RConn3
  HV Transformer 3/LConn1 -- Three-Phase PI Section Line16/LConn1 -- Three-Phase PI Section Line5/LConn1 -- Three-Phase PI Section Line15/RConn1 -- Three-Phase PI Section Line4/RConn1 -- HV Transformer 2/LConn1 -- Load Flow Bus2/RConn1
  Load Flow Bus2/LConn2 -- HV Source 2/RConn2
  Load Flow Bus2/LConn1 -- HV Source 2/RConn1
  Load Flow Bus3/RConn1 -- Three-Phase V-I Measurement3/LConn1
  Load Flow Bus3/RConn2 -- Three-Phase V-I Measurement3/LConn2
  Load Flow Bus3/RConn3 -- Three-Phase V-I Measurement3/LConn3
  Load Flow Bus4/RConn1 -- Three-Phase V-I Measurement1/LConn1
  Load Flow Bus4/RConn2 -- Three-Phase V-I Measurement1/LConn2
  Load Flow Bus4/RConn3 -- Three-Phase V-I Measurement1/LConn3
  Load Flow Bus5/RConn1 -- Three-Phase V-I Measurement4/LConn1
  Load Flow Bus5/RConn2 -- Three-Phase V-I Measurement4/LConn2
  Load Flow Bus5/RConn3 -- Three-Phase V-I Measurement4/LConn3
  Load Flow Bus6/RConn1 -- Three-Phase V-I Measurement6/LConn1
  Load Flow Bus6/RConn2 -- Three-Phase V-I Measurement6/LConn2
  Load Flow Bus6/RConn3 -- Three-Phase V-I Measurement6/LConn3
  Load Flow Bus7/RConn1 -- Three-Phase V-I Measurement7/LConn1
  Load Flow Bus7/RConn2 -- Three-Phase V-I Measurement7/LConn2
  Load Flow Bus7/RConn3 -- Three-Phase V-I Measurement7/LConn3
  Load Flow Bus8/RConn1 -- Three-Phase V-I Measurement8/LConn1
  Load Flow Bus8/RConn2 -- Three-Phase V-I Measurement8/LConn2
  Load Flow Bus8/RConn3 -- Three-Phase V-I Measurement8/LConn3
  Load Flow Bus9/RConn1 -- Three-Phase V-I Measurement9/LConn1
  Load Flow Bus9/RConn2 -- Three-Phase V-I Measurement9/LConn2
  Load Flow Bus9/RConn3 -- Three-Phase V-I Measurement9/LConn3
  Load Flow Bus14/RConn1 -- Three-Phase V-I Measurement5/LConn1
  Load Flow Bus14/RConn2 -- Three-Phase V-I Measurement5/LConn2
  Load Flow Bus14/RConn3 -- Three-Phase V-I Measurement5/LConn3
  Load Flow Bus16/RConn1 -- Three-Phase V-I Measurement2/LConn1
  Load Flow Bus16/RConn2 -- Three-Phase V-I Measurement2/LConn2
  Load Flow Bus16/RConn3 -- Three-Phase V-I Measurement2/LConn3
  Load Flow Bus/RConn1 -- Three-Phase PI Section Line17/LConn1 -- Three-Phase PI Section Line12/LConn1 -- Three-Phase PI Section Line4/LConn1 -- Three-Phase PI Section Line15/LConn1 -- " "/LConn1
  Load Flow Bus/LConn3 -- HV Source 1/RConn3
  Load Flow Bus/RConn2 -- Three-Phase PI Section Line17/LConn2 -- Three-Phase PI Section Line12/LConn2 -- Three-Phase PI Section Line4/LConn2 -- Three-Phase PI Section Line15/LConn2 -- " "/LConn2
  Three-Phase V-I Measurement10/RConn1 -- Three-Phase PI Section Line3/RConn1
  Three-Phase V-I Measurement10/RConn2 -- Three-Phase PI Section Line3/RConn2
  Three-Phase V-I Measurement10/RConn3 -- Three-Phase PI Section Line3/RConn3
  Three-Phase V-I Measurement10/LConn1 -- HV Transformer 2/RConn1
  Three-Phase V-I Measurement10/LConn2 -- HV Transformer 2/RConn2
  Three-Phase V-I Measurement10/LConn3 -- HV Transformer 2/RConn3
  Ground2/LConn1 -- Impedance Measurement/LConn2
  Three-Phase PI Section Line8/LConn1 -- Impedance Measurement/LConn1 -- Three-Phase PI Section Line14/LConn1 -- Three-Phase PI Section Line13/RConn1 -- Load Flow Bus14/LConn1 -- Three-Phase PI Section Line7/RConn1 -- Three-Phase V-I Measurement/LConn1
  Three-Phase PI Section Line8/LConn2 -- Three-Phase PI Section Line14/LConn2 -- Three-Phase PI Section Line13/RConn2 -- Three-Phase PI Section Line7/RConn2 -- Load Flow Bus14/LConn2 -- Three-Phase V-I Measurement/LConn2
  Three-Phase PI Section Line7/LConn2 -- Three-Phase PI Section Line13/LConn2 -- HV Transformer 3/RConn2 -- Load Flow Bus16/LConn2 -- Subsystem1/RConn2 -- Three-Phase PI Section Line6/RConn2

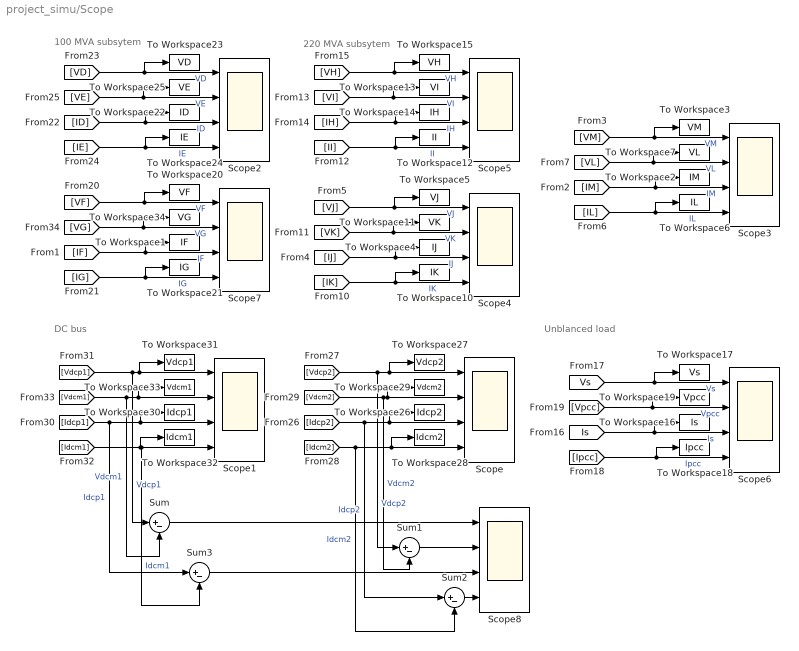
== system project_simu/Scope ==
  note: Unblanced load
  note: DC bus
  note: 220 MVA subsytem
  note: 100 MVA subsytem
  Scope{,1..8} (9 alike) : Scope  NumInputPorts=4
  Sum{,1..3} (4 alike) : Sum  Inputs=|+-
  To Workspace1 : ToWorkspace  VariableName=IF  SaveFormat=Timeseries  SampleTime=-1
  To Workspace10 : ToWorkspace  VariableName=IK  SaveFormat=Timeseries  SampleTime=-1
  To Workspace11 : ToWorkspace  VariableName=VK  SaveFormat=Timeseries  SampleTime=-1
  To Workspace12 : ToWorkspace  VariableName=II  SaveFormat=Timeseries  SampleTime=-1
  To Workspace13 : ToWorkspace  VariableName=VI  SaveFormat=Timeseries  SampleTime=-1
  To Workspace14 : ToWorkspace  VariableName=IH  SaveFormat=Timeseries  SampleTime=-1
  To Workspace15 : ToWorkspace  VariableName=VH  SaveFormat=Timeseries  SampleTime=-1
  To Workspace16 : ToWorkspace  VariableName=Is  SaveFormat=Timeseries  SampleTime=-1
  To Workspace17 : ToWorkspace  VariableName=Vs  SaveFormat=Timeseries  SampleTime=-1
  To Workspace18 : ToWorkspace  VariableName=Ipcc  SaveFormat=Timeseries  SampleTime=-1
  To Workspace19 : ToWorkspace  VariableName=Vpcc  SaveFormat=Timeseries  SampleTime=-1
  To Workspace2 : ToWorkspace  VariableName=IM  SaveFormat=Timeseries  SampleTime=-1
  To Workspace20 : ToWorkspace  VariableName=VF  SaveFormat=Timeseries  SampleTime=-1
  To Workspace21 : ToWorkspace  VariableName=IG  SaveFormat=Timeseries  SampleTime=-1
  To Workspace22 : ToWorkspace  VariableName=ID  SaveFormat=Timeseries  SampleTime=-1
  To Workspace23 : ToWorkspace  VariableName=VD  SaveFormat=Timeseries  SampleTime=-1
  To Workspace24 : ToWorkspace  VariableName=IE  SaveFormat=Timeseries  SampleTime=-1
  To Workspace25 : ToWorkspace  VariableName=VE  SaveFormat=Timeseries  SampleTime=-1
  To Workspace26 : ToWorkspace  VariableName=Idcp2  SaveFormat=Timeseries  SampleTime=-1
  To Workspace27 : ToWorkspace  VariableName=Vdcp2  SaveFormat=Timeseries  SampleTime=-1
  To Workspace28 : ToWorkspace  VariableName=Idcm2  SaveFormat=Timeseries  SampleTime=-1
  To Workspace29 : ToWorkspace  VariableName=Vdcm2  SaveFormat=Timeseries  SampleTime=-1
  To Workspace3 : ToWorkspace  VariableName=VM  SaveFormat=Timeseries  SampleTime=-1
  To Workspace30 : ToWorkspace  VariableName=Idcp1  SaveFormat=Timeseries  SampleTime=-1
  To Workspace31 : ToWorkspace  VariableName=Vdcp1  SaveFormat=Timeseries  SampleTime=-1
  To Workspace32 : ToWorkspace  VariableName=Idcm1  SaveFormat=Timeseries  SampleTime=-1
  To Workspace33 : ToWorkspace  VariableName=Vdcm1  SaveFormat=Timeseries  SampleTime=-1
  To Workspace34 : ToWorkspace  VariableName=VG  SaveFormat=Timeseries  SampleTime=-1
  To Workspace4 : ToWorkspace  VariableName=IJ  SaveFormat=Timeseries  SampleTime=-1
  To Workspace5 : ToWorkspace  VariableName=VJ  SaveFormat=Timeseries  SampleTime=-1
  To Workspace6 : ToWorkspace  VariableName=IL  SaveFormat=Timeseries  SampleTime=-1
  To Workspace7 : ToWorkspace  VariableName=VL  SaveFormat=Timeseries  SampleTime=-1
  wires:
  [VI] -> To Workspace13/1, Scope5/2  "VI"
  [VF] -> To Workspace20/1, Scope7/1  "VF"
  [Idcp1] -> Sum3/1, Scope1/3, To Workspace30/1  "Idcp1"
  [IG] -> Scope7/4, To Workspace21/1  "IG"
  [IE] -> Scope2/4, To Workspace24/1  "IE"
  [Vdcm2] -> Scope/2, To Workspace29/1, Sum1/2  "Vdcm2"
  [VM] -> To Workspace3/1, Scope3/1  "VM"
  [IF] -> Scope7/3, To Workspace1/1  "IF"
  [Vdcp1] -> Sum/1, To Workspace31/1, Scope1/1  "Vdcp1"
  [VH] -> To Workspace15/1, Scope5/1  "VH"
  [IM] -> Scope3/3, To Workspace2/1  "IM"
  [VG] -> To Workspace34/1, Scope7/2  "VG"
  [Vs] -> To Workspace17/1, Scope6/1  "Vs"
  [IL] -> Scope3/4, To Workspace6/1  "IL"
  [II] -> Scope5/4, To Workspace12/1  "II"
  [IJ] -> Scope4/3, To Workspace4/1  "IJ"
  [Vdcp2] -> Sum1/1, To Workspace27/1, Scope/1  "Vdcp2"
  [IH] -> Scope5/3, To Workspace14/1  "IH"
  [Ipcc] -> To Workspace18/1, Scope6/4  "Ipcc"
  [Vpcc] -> To Workspace19/1, Scope6/2  "Vpcc"
  [VJ] -> To Workspace5/1, Scope4/1  "VJ"
  [Vdcm1] -> Sum/2, To Workspace33/1, Scope1/2  "Vdcm1"
  [IK] -> Scope4/4, To Workspace10/1  "IK"
  [VK] -> To Workspace11/1, Scope4/2  "VK"
  [VL] -> To Workspace7/1, Scope3/2  "VL"
  [Idcp2] -> Sum2/1, Scope/3, To Workspace26/1  "Idcp2"
  [VD] -> To Workspace23/1, Scope2/1  "VD"
  [Is] -> Scope6/3, To Workspace16/1  "Is"
  [Idcm1] -> Sum3/2, Scope1/4, To Workspace32/1  "Idcm1"
  [ID] -> Scope2/3, To Workspace22/1  "ID"
  [Idcm2] -> Sum2/2, To Workspace28/1, Scope/4  "Idcm2"
  [VE] -> To Workspace25/1, Scope2/2  "VE"
  Sum/1 -> Scope8/1
  Sum1/1 -> Scope8/2
  Sum3/1 -> Scope8/3
  Sum2/1 -> Scope8/4
